simulink model "PID"  (R2023b)
settings: Solver=VariableStepAuto  StartTime=0.0  StopTime=50  RelTol=1e-3
settings Model: Creator=nocto  LastModifiedBy=nocto

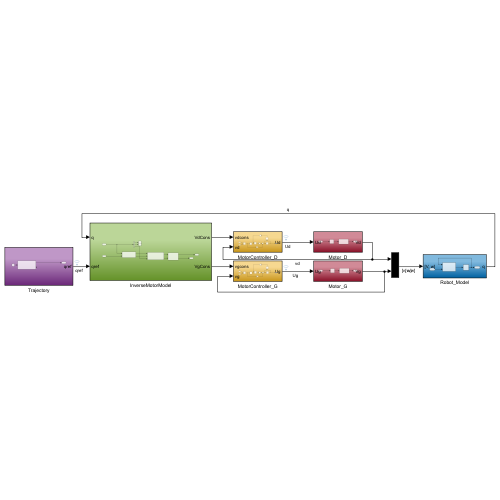
[thumbnail: Simulink's stored preview of the top-level diagram]
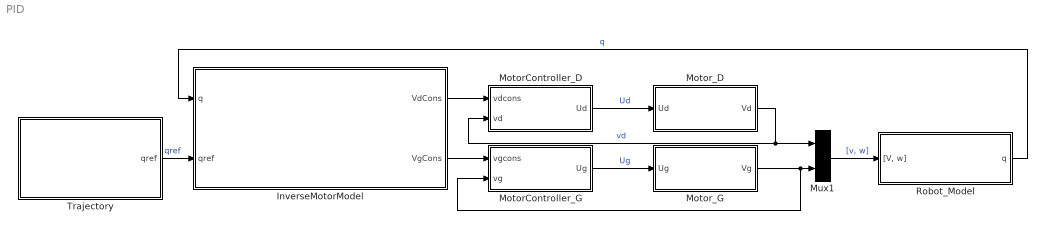
== system PID ==
  InverseMotorModel : Subsystem
  MotorController_D : Subsystem
  MotorController_G : Subsystem
  Motor_D : Subsystem
  Motor_G : Subsystem
  Mux1 : Mux  Inputs=2
  Robot_Model : Subsystem
  Trajectory : Subsystem
  wires:
  Robot_Model/1(q) -> InverseMotorModel/1(q)  "q"
  Trajectory/1(qref) -> InverseMotorModel/2(qref)  "qref"
  Motor_D/1(Vd) -> MotorController_D/2(vd), Mux1/1  "vd"
  Motor_G/1(Vg) -> MotorController_G/2(vg), Mux1/2
  Mux1/1 -> Robot_Model/1("[V, w]")  "[v, w]"
  InverseMotorModel/1(VdCons) -> MotorController_D/1(vdcons)
  InverseMotorModel/2(VgCons) -> MotorController_G/1(vgcons)
  MotorController_G/1(Ug) -> Motor_G/1(Ug)  "Ug"
  MotorController_D/1(Ud) -> Motor_D/1(Ud)  "Ud"

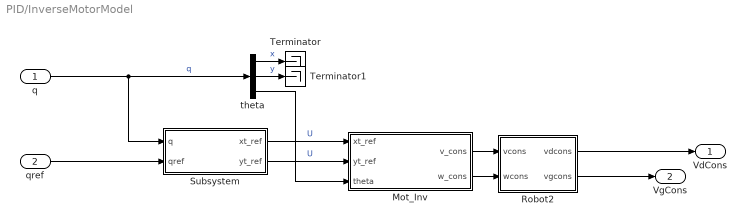
== system PID/InverseMotorModel ==
  q : Inport
  qref : Inport  Port=2
  Mot_Inv : MATLAB Function  TreatAsAtomicUnit=on
  Robot2 : MATLAB Function  TreatAsAtomicUnit=on
  Subsystem : Subsystem
  Terminator : Terminator
  Terminator1 : Terminator
  theta : Demux  Outputs=3
  VdCons : Outport
  VgCons : Outport  Port=2
  wires:
  theta/2 -> Terminator1/1  "y"
  Subsystem/2(yt_ref) -> Mot_Inv/2(yt_ref)  "U"
  Subsystem/1(xt_ref) -> Mot_Inv/1(xt_ref)  "U"
  q/1 -> Subsystem/1(q), theta/1  "q"
  Mot_Inv/2(w_cons) -> Robot2/2(wcons)
  theta/1 -> Terminator/1  "x"
  theta/3 -> Mot_Inv/3(theta)
  Mot_Inv/1(v_cons) -> Robot2/1(vcons)
  qref/1 -> Subsystem/2(qref)
  Robot2/2(vgcons) -> VgCons/1
  Robot2/1(vdcons) -> VdCons/1

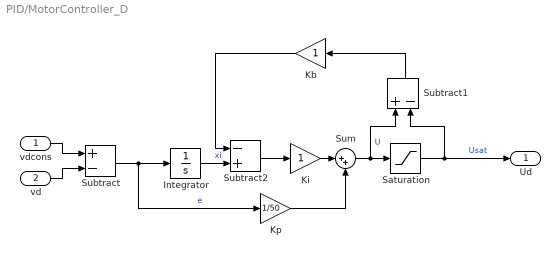
== system PID/MotorController_D ==
  vdcons : Inport
  vd : Inport  Port=2
  Integrator : Integrator
  Kb : Gain
  Ki : Gain
  Kp : Gain  Gain=1/50
  Saturation : Saturate  UpperLimit=4.5  LowerLimit=-4.5
  Subtract : Sum  Inputs=+-
  Subtract1 : Sum  Inputs=+-
  Subtract2 : Sum  Inputs=-+
  Sum : Sum  Inputs=|++
  Ud : Outport
  wires:
  Subtract1/1 -> Kb/1
  Integrator/1 -> Subtract2/2  "xi"
  Kb/1 -> Subtract2/1
  Kp/1 -> Sum/2
  Sum/1 -> Saturation/1, Subtract1/1  "U"
  Saturation/1 -> Ud/1, Subtract1/2  "Usat"
  Subtract2/1 -> Ki/1
  vdcons/1 -> Subtract/1
  vd/1 -> Subtract/2
  Subtract/1 -> Kp/1, Integrator/1  "e"
  Ki/1 -> Sum/1

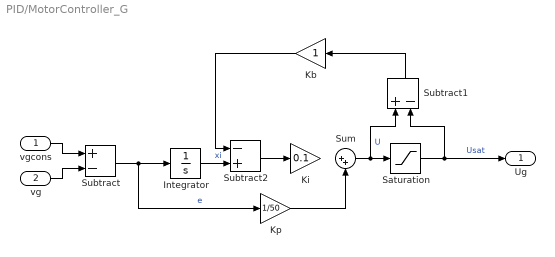
== system PID/MotorController_G ==
  vgcons : Inport
  vg : Inport  Port=2
  Integrator : Integrator
  Kb : Gain
  Ki : Gain  Gain=0.1
  Kp : Gain  Gain=1/50
  Saturation : Saturate  UpperLimit=4.5  LowerLimit=-4.5
  Subtract : Sum  Inputs=+-
  Subtract1 : Sum  Inputs=+-
  Subtract2 : Sum  Inputs=-+
  Sum : Sum  Inputs=|++
  Ug : Outport
  wires:
  Subtract/1 -> Integrator/1, Kp/1  "e"
  vg/1 -> Subtract/2
  vgcons/1 -> Subtract/1
  Subtract2/1 -> Ki/1
  Saturation/1 -> Ug/1, Subtract1/2  "Usat"
  Sum/1 -> Subtract1/1, Saturation/1  "U"
  Kp/1 -> Sum/2
  Kb/1 -> Subtract2/1
  Integrator/1 -> Subtract2/2  "xi"
  Subtract1/1 -> Kb/1

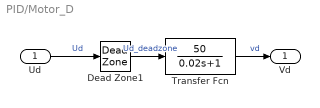
== system PID/Motor_D ==
  Ud : Inport
  Dead Zone1 : DeadZone  LowerValue=-1  UpperValue=1
  Transfer Fcn : TransferFcn  Numerator=[50]  Denominator=[0.02 1]
  Vd : Outport
  wires:
  Dead Zone1/1 -> Transfer Fcn/1  "Ud_deadzone"
  Ud/1 -> Dead Zone1/1  "Ud"
  Transfer Fcn/1 -> Vd/1  "vd"

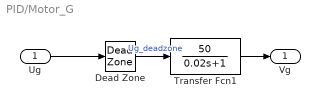
== system PID/Motor_G ==
  Ug : Inport
  Dead Zone : DeadZone
  Transfer Fcn1 : TransferFcn  Numerator=[50]  Denominator=[0.02 1]
  Vg : Outport
  wires:
  Dead Zone/1 -> Transfer Fcn1/1  "Ug_deadzone"
  Transfer Fcn1/1 -> Vg/1
  Ug/1 -> Dead Zone/1

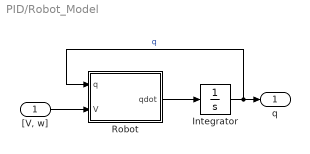
== system PID/Robot_Model ==
  "[V, w]" : Inport
  Integrator : Integrator  InitialCondition=[0; 0; 0]
  Robot : MATLAB Function  TreatAsAtomicUnit=on
  q : Outport
  wires:
  Robot/1(qdot) -> Integrator/1
  "[V, w]"/1 -> Robot/2(V)
  Integrator/1 -> Robot/1(q), q/1  "q"

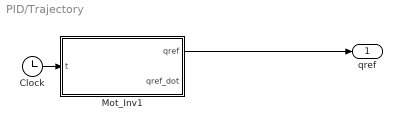
== system PID/Trajectory ==
  Clock : Clock
  Mot_Inv1 : MATLAB Function  TreatAsAtomicUnit=on
  qref : Outport
  wires:
  Mot_Inv1/1(qref) -> qref/1
  Clock/1 -> Mot_Inv1/1(t)

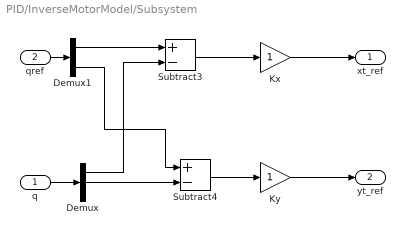
== system PID/InverseMotorModel/Subsystem ==
  q : Inport
  qref : Inport  Port=2
  Demux : Demux  Outputs=3
  Demux1 : Demux  Outputs=2
  Kx : Gain
  Ky : Gain
  Subtract3 : Sum  Inputs=+-
  Subtract4 : Sum  Inputs=+-
  xt_ref : Outport
  yt_ref : Outport  Port=2
  wires:
  q/1 -> Demux/1
  Demux/1 -> Subtract3/2
  Demux/2 -> Subtract4/2
  qref/1 -> Demux1/1
  Demux1/1 -> Subtract3/1
  Subtract3/1 -> Kx/1
  Demux1/2 -> Subtract4/1
  Subtract4/1 -> Ky/1
  Ky/1 -> yt_ref/1
  Kx/1 -> xt_ref/1

== matlab function PID/Trajectory/Mot_Inv1 ==
  data: t input; qref output; qref_dot output
function [qref, qref_dot]= Polynomial(t)
X = [0; 300; 0; 0];
Y = [0; -750; 0; 0];

t0 = 0;
tf = 25;
lambda = (t-t0)/(tf-t0);

a0 = X(1); a1 = (tf-t0)*X(3);
a3 = (tf-t0)*(X(4) + X(3)) + 2*(X(1) - X(2));
a2 = X(2) - a0 - a1 - a3;

b0 = Y(1); b1 = (tf-t0)*Y(3);
b3 = (tf-t0)*(Y(4) + Y(3)) + 2*(Y(1) - Y(2));
b2 = Y(2) - b0 - b1 - b3;

if t < tf
    qref = [a0 + a1*lambda + a2*lambda^2 + a3*lambda^3;
    b0 + b1*lambda + b2*lambda^2 + b3*lambda^3];

    qref_dot = [a1 + 2*a2*lambda + a3*lambda^2;
        b1 + 2*b2*lambda + b3*lambda^2]/(tf-t0);
else
    qref = [X(2); Y(2)];
    qref_dot = [0;
        0];
end

== matlab function PID/Robot_Model/Robot ==
  data: q input; qdot output; V input
function qdot = RobotModel(q, V)
qdot = zeros(3, 1);
l = 90;
L = 115;

v = (V(1) + V(2))/2;
w = (V(1) - V(2))/(2*l);

qdot(1) = v*cos(q(3)) - w*L*sin(q(3));
qdot(2) = v*sin(q(3)) + w*L*cos(q(3));
qdot(3) = w;

== matlab function PID/InverseMotorModel/Robot2 ==
  data: vcons input; vdcons output; wcons input; vgcons output
function [vdcons, vgcons] = WheelsToRobot(vcons, wcons)
l = 90;

vdcons = vcons + l * wcons;
vgcons = vcons - l * wcons;

== matlab function PID/InverseMotorModel/Mot_Inv ==
  data: xt_ref input; v_cons output; yt_ref input; w_cons output; theta input
function [v_cons, w_cons] = fcn(xt_ref, yt_ref, theta)
l = 90;
L = 115;

A = [cos(theta) -L*sin(theta);
    sin(theta) L*cos(theta)];

V = A\[xt_ref; yt_ref];
v_cons = V(1); w_cons = V(2);
